simulink model "generic_20250508_0051_updated"  (R2024a)
settings: Solver=FixedStepDiscrete  StartTime=0.0  StopTime=inf  FixedStep=0.001  RelTol=1e-3  EnableMultiTasking=on
undefined symbols (not defined in the file): left_first_line_point_x, right_first_line_point_x, route1_waypoint_raw
libraries: CarMaker4SL x62, slpidlib x3, simulink x1
(part 3 of 3)

== system generic_20250508_0051_updated/CarMaker/IPG Vehicle/CarAndTrailer/Forces/Vehicle Forces ==
  Sync_In : Inport
  Bus Creator1 : BusCreator  Inputs=12
  Bus Creator8 : BusCreator  Inputs=16
  BusCreator1 : BusCreator  Inputs=4
  BusCreator2 : BusCreator  Inputs=9
  Demux : Demux  Outputs=16
      settings: DisplayOption=none
  Demux1 : Demux  Outputs=12
      settings: DisplayOption=none
  Demux2 : Demux  Outputs=13
      settings: DisplayOption=none
  Forces : S-Function  FunctionName=CM_Sfun  Parameters='Forces'  SFunctionDeploymentMode=off  EnableBusSupport=off
  Terminator : Terminator
  Sync_Out : Outport  VectorParamsAs1DForOutWhenUnconnected=off
  Car.Virtual : Outport  Port=2  VectorParamsAs1DForOutWhenUnconnected=off
  Car.Aero : Outport  Port=3  VectorParamsAs1DForOutWhenUnconnected=off
  Car.Load : Outport  Port=4  VectorParamsAs1DForOutWhenUnconnected=off
  wires:
  BusCreator1/1 -> Terminator/1  "Aero IF (in)"
  Demux2/13 -> BusCreator2/9  "car Aero Trq_1 z"
  Demux2/12 -> BusCreator2/8  "car Aero Trq_1 y"
  Demux2/11 -> BusCreator2/7  "car Aero Trq_1 x"
  Demux2/10 -> BusCreator2/6  "car Aero Frc_1 z"
  Demux2/9 -> BusCreator2/5  "car Aero Frc_1 y"
  Demux2/8 -> BusCreator2/4  "car Aero Frc_1 x"
  Demux2/7 -> BusCreator2/3  "car Aero PoA_1 z"
  Demux2/6 -> BusCreator2/2  "car Aero PoA_1 y"
  Demux2/5 -> BusCreator2/1  "car Aero PoA_1 x"
  Demux2/4 -> BusCreator1/4  "car Aero tau_1"
  Demux2/3 -> BusCreator1/3  "car Aero ApproachVel_1 z"
  Demux2/2 -> BusCreator1/2  "car Aero ApproachVel_1 y"
  Demux2/1 -> BusCreator1/1  "car Aero ApproachVel_1 x"
  Demux/16 -> Bus Creator8/16  "Car Load_3 tz"
  Demux/15 -> Bus Creator8/15  "Car Load_3 ty"
  Demux/14 -> Bus Creator8/14  "Car Load_3 tx"
  Demux/13 -> Bus Creator8/13  "Car Load_3 mass"
  Demux1/12 -> Bus Creator1/12  "Car Virtual Trq_0 z"
  Demux1/11 -> Bus Creator1/11  "Car Virtual Trq_0 y"
  Demux1/10 -> Bus Creator1/10  "Car Virtual Trq_0 x"
  Demux1/9 -> Bus Creator1/9  "Car Virtual Trq_1 z"
  Demux1/8 -> Bus Creator1/8  "Car Virtual Trq_1 y"
  Demux1/7 -> Bus Creator1/7  "Car Virtual Trq_1 x"
  Demux1/6 -> Bus Creator1/6  "Car Virtual Frc_0 z"
  Demux1/5 -> Bus Creator1/5  "Car Virtual Frc_0 y"
  Demux1/4 -> Bus Creator1/4  "Car Virtual Frc_0 x"
  Sync_In/1 -> Forces/1
  Forces/1 -> Sync_Out/1
  BusCreator2/1 -> Car.Aero/1
  Demux1/1 -> Bus Creator1/1  "Car Virtual Frc_1 x"
  Demux1/2 -> Bus Creator1/2  "Car Virtual Frc_1 y"
  Demux1/3 -> Bus Creator1/3  "Car Virtual Frc_1 z"
  Forces/3 -> Demux2/1
  Forces/2 -> Demux1/1
  Bus Creator1/1 -> Car.Virtual/1
  Bus Creator8/1 -> Car.Load/1
  Demux/1 -> Bus Creator8/1  "Car Load_0 mass"
  Demux/2 -> Bus Creator8/2  "Car Load_0 tx"
  Demux/3 -> Bus Creator8/3  "Car Load_0 ty"
  Demux/4 -> Bus Creator8/4  "Car Load_0 tz"
  Demux/5 -> Bus Creator8/5  "Car Load_1 mass"
  Demux/6 -> Bus Creator8/6  "Car Load_1 tx"
  Demux/7 -> Bus Creator8/7  "Car Load_1 ty"
  Demux/8 -> Bus Creator8/8  "Car Load_1 tz"
  Demux/9 -> Bus Creator8/9  "Car Load_2 mass"
  Demux/10 -> Bus Creator8/10  "Car Load_2 tx"
  Demux/11 -> Bus Creator8/11  "Car Load_2 ty"
  Demux/12 -> Bus Creator8/12  "Car Load_2 tz"
  Forces/4 -> Demux/1

== system generic_20250508_0051_updated/CarMaker/IPG Vehicle/CarAndTrailer/Trailer/CreateBus Car.Hitch.FrcTrq ==
  In1 : Inport
  Bus Creator7 : BusCreator  Inputs=6
  Demux7 : Demux  Outputs=6
      settings: DisplayOption=none
  Out1 : Outport  VectorParamsAs1DForOutWhenUnconnected=off
  wires:
  In1/1 -> Demux7/1
  Bus Creator7/1 -> Out1/1
  Demux7/6 -> Bus Creator7/6  "Car Hitch Trq2Car z"
  Demux7/5 -> Bus Creator7/5  "Car Hitch Trq2Car y"
  Demux7/4 -> Bus Creator7/4  "Car Hitch Trq2Car x"
  Demux7/3 -> Bus Creator7/3  "Car Hitch Frc2Car z"
  Demux7/2 -> Bus Creator7/2  "Car Hitch Frc2Car y"
  Demux7/1 -> Bus Creator7/1  "Car Hitch Frc2Car x"

== system generic_20250508_0051_updated/CarMaker/IPG Vehicle/CarAndTrailer/Trailer/CreateBus Vhcl.Motion ==
  In1 : Inport
  BusCreator : BusCreator  Inputs=15
  Demux : Demux  Outputs=15
      settings: DisplayOption=none
  Out1 : Outport  VectorParamsAs1DForOutWhenUnconnected=off
  wires:
  Demux/15 -> BusCreator/15  "Vhcl YawAcc"
  Demux/14 -> BusCreator/14  "Vhcl YawVel"
  Demux/13 -> BusCreator/13  "Vhcl Yaw"
  Demux/12 -> BusCreator/12  "Vhcl PitchAcc"
  Demux/11 -> BusCreator/11  "Vhcl PitchVel"
  Demux/10 -> BusCreator/10  "Vhcl Pitch"
  Demux/9 -> BusCreator/9  "Vhcl RollAcc"
  Demux/8 -> BusCreator/8  "Vhcl RollVel"
  Demux/7 -> BusCreator/7  "Vhcl Roll"
  Demux/6 -> BusCreator/6  "Vhcl Hitch_Pos z"
  Demux/5 -> BusCreator/5  "Vhcl Hitch_Pos y"
  Demux/4 -> BusCreator/4  "Vhcl Hitch_Pos x"
  Demux/3 -> BusCreator/3  "Vhcl sRoad"
  Demux/2 -> BusCreator/2  "Vhcl Distance"
  Demux/1 -> BusCreator/1  "Vhcl v"
  In1/1 -> Demux/1
  BusCreator/1 -> Out1/1

== system generic_20250508_0051_updated/CarMaker/IPG Vehicle/CarAndTrailer/Trailer/CreateBus Vhcl.PoI ==
  In1 : Inport
  Bus Creator3 : BusCreator  Inputs=18
  Demux3 : Demux  Outputs=18
      settings: DisplayOption=none
  Out1 : Outport  VectorParamsAs1DForOutWhenUnconnected=off
  wires:
  Demux3/18 -> Bus Creator3/18  "Vhcl PoI_GCS Elev"
  Demux3/17 -> Bus Creator3/17  "Vhcl PoI_GCS Lat"
  Demux3/16 -> Bus Creator3/16  "Vhcl PoI_GCS Long"
  Demux3/15 -> Bus Creator3/15  "Vhcl PoI_Acc_1 z"
  Demux3/14 -> Bus Creator3/14  "Vhcl PoI_Acc_1 y"
  Demux3/13 -> Bus Creator3/13  "Vhcl PoI_Acc_1 x"
  Demux3/12 -> Bus Creator3/12  "Vhcl PoI_Vel_1 z"
  Demux3/11 -> Bus Creator3/11  "Vhcl PoI_Vel_1 y"
  Demux3/10 -> Bus Creator3/10  "Vhcl PoI_Vel_1 x"
  Demux3/9 -> Bus Creator3/9  "Vhcl PoI_Acc z"
  Demux3/8 -> Bus Creator3/8  "Vhcl PoI_Acc y"
  Demux3/7 -> Bus Creator3/7  "Vhcl PoI_Acc x"
  Demux3/6 -> Bus Creator3/6  "Vhcl PoI_Vel z"
  Demux3/5 -> Bus Creator3/5  "Vhcl PoI_Vel y"
  Demux3/4 -> Bus Creator3/4  "Vhcl PoI_Vel x"
  Demux3/3 -> Bus Creator3/3  "Vhcl PoI_Pos z"
  Demux3/2 -> Bus Creator3/2  "Vhcl PoI_Pos y"
  In1/1 -> Demux3/1
  Bus Creator3/1 -> Out1/1
  Demux3/1 -> Bus Creator3/1  "Vhcl PoI_Pos x"

== system generic_20250508_0051_updated/CarMaker/IPG Vehicle/CarAndTrailer/Trailer/CreateBus Vhcl.Steering ==
  In1 : Inport
  Bus Creator3 : BusCreator  Inputs=4
  Demux : Demux
      settings: DisplayOption=none
  Out1 : Outport  VectorParamsAs1DForOutWhenUnconnected=off
  wires:
  Bus Creator3/1 -> Out1/1
  Demux/1 -> Bus Creator3/1  "Vhcl Steering Ang"
  Demux/3 -> Bus Creator3/3  "Vhcl Steering AngAcc"
  Demux/2 -> Bus Creator3/2  "Vhcl Steering AngVel"
  Demux/4 -> Bus Creator3/4  "Vhcl Steering Trq"
  In1/1 -> Demux/1

== system generic_20250508_0051_updated/CarMaker/IPG Vehicle/CarAndTrailer/Trailer/CreateBus Vhcl.Wheel.FL ==
  In1 : Inport
  Bus Creator3 : BusCreator  Inputs=14
  Demux3 : Demux  Outputs=14
      settings: DisplayOption=none
  Out1 : Outport  VectorParamsAs1DForOutWhenUnconnected=off
  wires:
  Demux3/14 -> Bus Creator3/14  "Vhcl Wheel FL Trq_WhlBearing"
  Demux3/13 -> Bus Creator3/13  "Vhcl Wheel FL Trq_T2W"
  Demux3/12 -> Bus Creator3/12  "Vhcl Wheel FL SideSlip"
  Demux3/11 -> Bus Creator3/11  "Vhcl Wheel FL LongSlip"
  Demux3/10 -> Bus Creator3/10  "Vhcl Wheel FL vBelt"
  Demux3/9 -> Bus Creator3/9  "Vhcl Wheel FL Fz"
  Demux3/8 -> Bus Creator3/8  "Vhcl Wheel FL Fy"
  Demux3/7 -> Bus Creator3/7  "Vhcl Wheel FL Fx"
  Demux3/6 -> Bus Creator3/6  "Vhcl Wheel FL r_zxy z"
  Demux3/5 -> Bus Creator3/5  "Vhcl Wheel FL r_zxy y"
  Demux3/4 -> Bus Creator3/4  "Vhcl Wheel FL r_zxy x"
  Demux3/3 -> Bus Creator3/3  "Vhcl Wheel FL t z"
  Demux3/2 -> Bus Creator3/2  "Vhcl Wheel FL t y"
  In1/1 -> Demux3/1
  Bus Creator3/1 -> Out1/1
  Demux3/1 -> Bus Creator3/1  "Vhcl Wheel FL t x"

== system generic_20250508_0051_updated/CarMaker/IPG Vehicle/CarAndTrailer/Trailer/CreateBus Vhcl.Wheel.FR ==
  In1 : Inport
  Bus Creator3 : BusCreator  Inputs=14
  Demux3 : Demux  Outputs=14
      settings: DisplayOption=none
  Out1 : Outport  VectorParamsAs1DForOutWhenUnconnected=off
  wires:
  Demux3/14 -> Bus Creator3/14  "Vhcl Wheel FR Trq_WhlBearing"
  Demux3/13 -> Bus Creator3/13  "Vhcl Wheel FR Trq_T2W"
  Demux3/12 -> Bus Creator3/12  "Vhcl Wheel FR SideSlip"
  Demux3/11 -> Bus Creator3/11  "Vhcl Wheel FR LongSlip"
  Demux3/10 -> Bus Creator3/10  "Vhcl Wheel FR vBelt"
  Demux3/9 -> Bus Creator3/9  "Vhcl Wheel FR Fz"
  Demux3/8 -> Bus Creator3/8  "Vhcl Wheel FR Fy"
  Demux3/7 -> Bus Creator3/7  "Vhcl Wheel FR Fx"
  Demux3/6 -> Bus Creator3/6  "Vhcl Wheel FR r_zxy z"
  Demux3/5 -> Bus Creator3/5  "Vhcl Wheel FR r_zxy y"
  Demux3/4 -> Bus Creator3/4  "Vhcl Wheel FR r_zxy x"
  Demux3/3 -> Bus Creator3/3  "Vhcl Wheel FR t z"
  Demux3/2 -> Bus Creator3/2  "Vhcl Wheel FR t y"
  In1/1 -> Demux3/1
  Bus Creator3/1 -> Out1/1
  Demux3/1 -> Bus Creator3/1  "Vhcl Wheel FR t x"

== system generic_20250508_0051_updated/CarMaker/IPG Vehicle/CarAndTrailer/Trailer/CreateBus Vhcl.Wheel.RL ==
  In1 : Inport
  Bus Creator3 : BusCreator  Inputs=14
  Demux3 : Demux  Outputs=14
      settings: DisplayOption=none
  Out1 : Outport  VectorParamsAs1DForOutWhenUnconnected=off
  wires:
  Demux3/14 -> Bus Creator3/14  "Vhcl Wheel RL Trq_WhlBearing"
  Demux3/13 -> Bus Creator3/13  "Vhcl Wheel RL Trq_T2W"
  Demux3/12 -> Bus Creator3/12  "Vhcl Wheel RL SideSlip"
  Demux3/11 -> Bus Creator3/11  "Vhcl Wheel RL LongSlip"
  Demux3/10 -> Bus Creator3/10  "Vhcl Wheel RL vBelt"
  Demux3/9 -> Bus Creator3/9  "Vhcl Wheel RL Fz"
  Demux3/8 -> Bus Creator3/8  "Vhcl Wheel RL Fy"
  Demux3/7 -> Bus Creator3/7  "Vhcl Wheel RL Fx"
  Demux3/6 -> Bus Creator3/6  "Vhcl Wheel RL r_zxy z"
  Demux3/5 -> Bus Creator3/5  "Vhcl Wheel RL r_zxy y"
  Demux3/4 -> Bus Creator3/4  "Vhcl Wheel RL r_zxy x"
  Demux3/3 -> Bus Creator3/3  "Vhcl Wheel RL t z"
  Demux3/2 -> Bus Creator3/2  "Vhcl Wheel RL t y"
  In1/1 -> Demux3/1
  Bus Creator3/1 -> Out1/1
  Demux3/1 -> Bus Creator3/1  "Vhcl Wheel RL t x"

== system generic_20250508_0051_updated/CarMaker/IPG Vehicle/CarAndTrailer/Trailer/CreateBus Vhcl.Wheel.RR ==
  In1 : Inport
  Bus Creator3 : BusCreator  Inputs=14
  Demux3 : Demux  Outputs=14
      settings: DisplayOption=none
  Out1 : Outport  VectorParamsAs1DForOutWhenUnconnected=off
  wires:
  Demux3/14 -> Bus Creator3/14  "Vhcl Wheel RR Trq_WhlBearing"
  Demux3/13 -> Bus Creator3/13  "Vhcl Wheel RR Trq_T2W"
  Demux3/12 -> Bus Creator3/12  "Vhcl Wheel RR SideSlip"
  Demux3/11 -> Bus Creator3/11  "Vhcl Wheel RR LongSlip"
  Demux3/10 -> Bus Creator3/10  "Vhcl Wheel RR vBelt"
  Demux3/9 -> Bus Creator3/9  "Vhcl Wheel RR Fz"
  Demux3/8 -> Bus Creator3/8  "Vhcl Wheel RR Fy"
  Demux3/7 -> Bus Creator3/7  "Vhcl Wheel RR Fx"
  Demux3/6 -> Bus Creator3/6  "Vhcl Wheel RR r_zxy z"
  Demux3/5 -> Bus Creator3/5  "Vhcl Wheel RR r_zxy y"
  Demux3/4 -> Bus Creator3/4  "Vhcl Wheel RR r_zxy x"
  Demux3/3 -> Bus Creator3/3  "Vhcl Wheel RR t z"
  Demux3/2 -> Bus Creator3/2  "Vhcl Wheel RR t y"
  In1/1 -> Demux3/1
  Bus Creator3/1 -> Out1/1
  Demux3/1 -> Bus Creator3/1  "Vhcl Wheel RR t x"

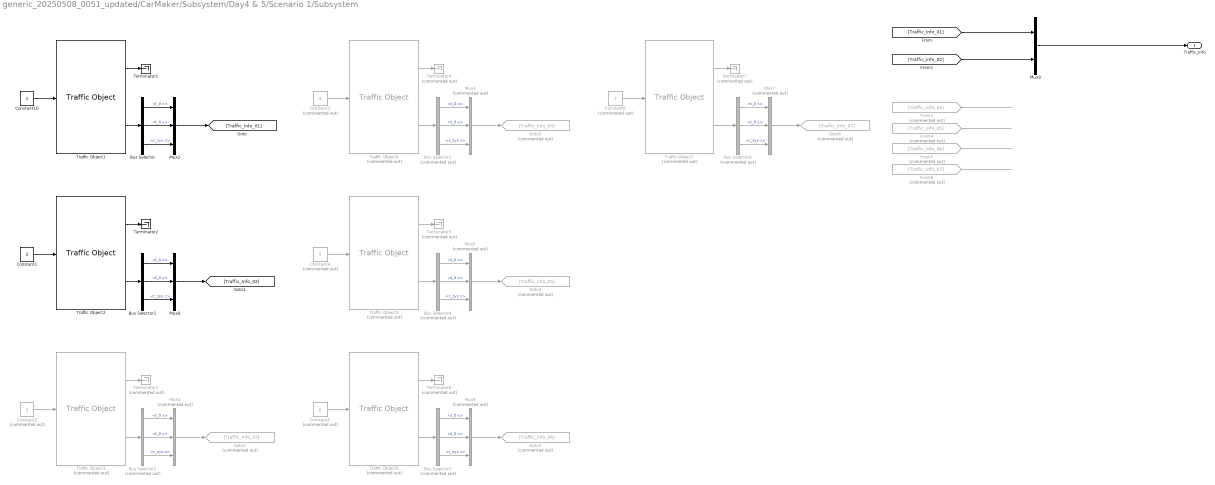
== system generic_20250508_0051_updated/CarMaker/Subsystem/Day4 & 5/Scenario 1/Subsystem ==
  Bus Selector : BusSelector  OutputSignals=t_0 x,t_0 y,r_zyx z
  Bus Selector1 : BusSelector  OutputSignals=t_0 x,t_0 y,r_zyx z
  Bus Selector{2..6} (5 alike) : BusSelector  Commented=on  OutputSignals=t_0 x,t_0 y,r_zyx z
  Constant1 : Constant  Value=2
  Constant10 : Constant
  Constant2 : Constant  Commented=on  Value=3
  Constant3 : Constant  Commented=on  Value=4
  Constant4 : Constant  Commented=on  Value=5
  Constant5 : Constant  Commented=on  Value=6
  Constant6 : Constant  Commented=on  Value=7
  From3 : From  Commented=on  GotoTag=Traffic_Info_04
  From4 : From  Commented=on  GotoTag=Traffic_Info_05
  From5 : From  Commented=on  GotoTag=Traffic_Info_06
  From6 : From  Commented=on  GotoTag=Traffic_Info_07
  Goto2 : Goto  Commented=on  GotoTag=Traffic_Info_03
  Goto3 : Goto  Commented=on  GotoTag=Traffic_Info_04
  Goto4 : Goto  Commented=on  GotoTag=Traffic_Info_05
  Goto5 : Goto  Commented=on  GotoTag=Traffic_Info_06
  Goto6 : Goto  Commented=on  GotoTag=Traffic_Info_07
  Mux2 : Mux  Inputs=3
  Mux{3..7} (5 alike) : Mux  Commented=on  Inputs=3
  Mux8 : Mux  Inputs=3
  Mux9 : Mux  Inputs=2
  Terminator1 : Terminator
  Terminator2 : Terminator
  Terminator{3..7} (5 alike) : Terminator  Commented=on
  Traffic Object1 : CarMaker4SL/Traffic Object  xname=T01  ximode=Traffic Id  xstime=Inherited
      settings: SourceProductName=CarMaker4SL
  Traffic Object2 : CarMaker4SL/Traffic Object  xname=T02  ximode=Traffic Id  xstime=Inherited
      settings: SourceProductName=CarMaker4SL
  Traffic Object3 : CarMaker4SL/Traffic Object  Commented=on  xname=T03  ximode=Traffic Id  xstime=Inherited
      settings: SourceProductName=CarMaker4SL
  Traffic Object4 : CarMaker4SL/Traffic Object  Commented=on  xname=T04  ximode=Traffic Id  xstime=Inherited
      settings: SourceProductName=CarMaker4SL
  Traffic Object5 : CarMaker4SL/Traffic Object  Commented=on  xname=T05  ximode=Traffic Id  xstime=Inherited
      settings: SourceProductName=CarMaker4SL
  Traffic Object6 : CarMaker4SL/Traffic Object  Commented=on  xname=T06  ximode=Traffic Id  xstime=Inherited
      settings: SourceProductName=CarMaker4SL
  Traffic Object7 : CarMaker4SL/Traffic Object  Commented=on  xname=T07  ximode=Traffic Id  xstime=Inherited
      settings: SourceProductName=CarMaker4SL
  Traffic_Info : Outport
  wires:
  Constant10/1 -> Traffic Object1/1
  Traffic Object1/1 -> Terminator1/1
  Traffic Object2/1 -> Terminator2/1
  Constant1/1 -> Traffic Object2/1
  Constant2/1 -> Traffic Object3/1
  Traffic Object3/1 -> Terminator3/1
  Traffic Object4/1 -> Terminator4/1
  Constant3/1 -> Traffic Object4/1
  Constant4/1 -> Traffic Object5/1
  Traffic Object5/1 -> Terminator5/1
  Traffic Object6/1 -> Terminator6/1
  Constant5/1 -> Traffic Object6/1
  Constant6/1 -> Traffic Object7/1
  Traffic Object7/1 -> Terminator7/1
  From3/1 -> ?
  From4/1 -> ?
  From5/1 -> ?
  From6/1 -> ?
  Traffic Object1/2 -> Bus Selector/1
  Bus Selector/1 -> Mux2/1  "<t_0 x>"
  Bus Selector/2 -> Mux2/2  "<t_0 y>"
  Bus Selector/3 -> Mux2/3  "<r_zyx z>"
  Bus Selector1/2 -> Mux8/2  "<t_0 y>"
  Mux8/1 -> [Traffic_Info_02]
  Bus Selector1/1 -> Mux8/1  "<t_0 x>"
  Bus Selector1/3 -> Mux8/3  "<r_zyx z>"
  Traffic Object2/2 -> Bus Selector1/1
  Bus Selector2/2 -> Mux3/2  "<t_0 y>"
  Mux3/1 -> Goto2/1
  Bus Selector2/1 -> Mux3/1  "<t_0 x>"
  Bus Selector2/3 -> Mux3/3  "<r_zyx z>"
  Traffic Object3/2 -> Bus Selector2/1
  Bus Selector3/2 -> Mux4/2  "<t_0 y>"
  Mux4/1 -> Goto3/1
  Bus Selector3/1 -> Mux4/1  "<t_0 x>"
  Bus Selector3/3 -> Mux4/3  "<r_zyx z>"
  Traffic Object4/2 -> Bus Selector3/1
  Bus Selector4/2 -> Mux5/2  "<t_0 y>"
  Mux5/1 -> Goto4/1
  Bus Selector4/1 -> Mux5/1  "<t_0 x>"
  Bus Selector4/3 -> Mux5/3  "<r_zyx z>"
  Traffic Object5/2 -> Bus Selector4/1
  Bus Selector5/2 -> Mux6/2  "<t_0 y>"
  Mux6/1 -> Goto5/1
  Bus Selector5/1 -> Mux6/1  "<t_0 x>"
  Bus Selector5/3 -> Mux6/3  "<r_zyx z>"
  Traffic Object6/2 -> Bus Selector5/1
  Bus Selector6/2 -> Mux7/2  "<t_0 y>"
  Mux7/1 -> Goto6/1
  Bus Selector6/1 -> Mux7/1  "<t_0 x>"
  Bus Selector6/3 -> Mux7/3  "<r_zyx z>"
  Traffic Object7/2 -> Bus Selector6/1
  Mux2/1 -> [Traffic_Info_01]
  [Traffic_Info_01] -> Mux9/1
  [Traffic_Info_02] -> Mux9/2
  Mux9/1 -> Traffic_Info/1

== system generic_20250508_0051_updated/CarMaker/IPG Vehicle/CarAndTrailer/Forces/Suspension Forces/Suspension External Forces Update ==
  Bus Creator21 : BusCreator  Inputs=6
  Bus Creator22 : BusCreator  Inputs=4
  Bus Creator23 : BusCreator  Inputs=4
  From : From  TagVisibility=global
  Ground{32..39} (8 alike) : Ground
  Out1 : Outport
  wires:
  [D] -> Bus Creator21/4
  Ground36/1 -> Bus Creator22/1
  From/1 -> Bus Creator21/1
  [B] -> Bus Creator21/2
  Ground34/1 -> Bus Creator23/3
  Ground32/1 -> Bus Creator23/1
  [C] -> Bus Creator21/3
  Bus Creator23/1 -> Bus Creator21/5
  Ground33/1 -> Bus Creator23/2
  Bus Creator22/1 -> Bus Creator21/6
  Bus Creator21/1 -> Out1/1
  Ground35/1 -> Bus Creator23/4
  Ground39/1 -> Bus Creator22/4
  Ground38/1 -> Bus Creator22/3
  Ground37/1 -> Bus Creator22/2

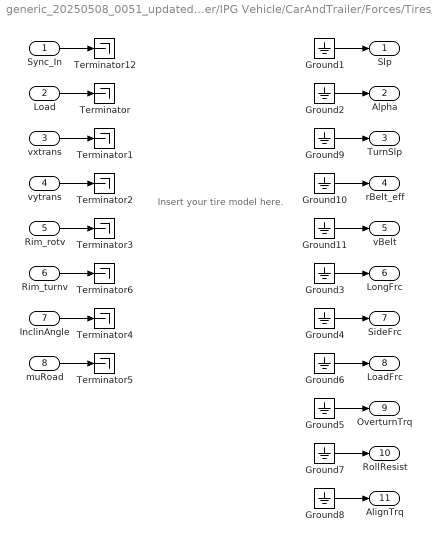
== system generic_20250508_0051_updated/CarMaker/IPG Vehicle/CarAndTrailer/Forces/Tires/TireFL ==
  note: Insert your tire model here.
  Sync_In : Inport
  Load : Inport  Port=2
  vxtrans : Inport  Port=3
  vytrans : Inport  Port=4
  Rim_rotv : Inport  Port=5
  Rim_turnv : Inport  Port=6
  InclinAngle : Inport  Port=7
  muRoad : Inport  Port=8
  Ground{1..11} (11 alike) : Ground
  Terminator{,1..6,12} (8 alike) : Terminator
  Slp : Outport  VectorParamsAs1DForOutWhenUnconnected=off
  Alpha : Outport  Port=2  VectorParamsAs1DForOutWhenUnconnected=off
  TurnSlp : Outport  Port=3  VectorParamsAs1DForOutWhenUnconnected=off
  rBelt_eff : Outport  Port=4  VectorParamsAs1DForOutWhenUnconnected=off
  vBelt : Outport  Port=5  VectorParamsAs1DForOutWhenUnconnected=off
  LongFrc : Outport  Port=6  VectorParamsAs1DForOutWhenUnconnected=off
  SideFrc : Outport  Port=7  VectorParamsAs1DForOutWhenUnconnected=off
  LoadFrc : Outport  Port=8  VectorParamsAs1DForOutWhenUnconnected=off
  OverturnTrq : Outport  Port=9  VectorParamsAs1DForOutWhenUnconnected=off
  RollResist : Outport  Port=10  VectorParamsAs1DForOutWhenUnconnected=off
  AlignTrq : Outport  Port=11  VectorParamsAs1DForOutWhenUnconnected=off
  wires:
  Ground11/1 -> vBelt/1
  Ground10/1 -> rBelt_eff/1
  Ground9/1 -> TurnSlp/1
  Rim_turnv/1 -> Terminator6/1
  Sync_In/1 -> Terminator12/1
  Ground2/1 -> Alpha/1
  Ground3/1 -> LongFrc/1
  Ground4/1 -> SideFrc/1
  Ground5/1 -> OverturnTrq/1
  vxtrans/1 -> Terminator1/1
  vytrans/1 -> Terminator2/1
  Rim_rotv/1 -> Terminator3/1
  InclinAngle/1 -> Terminator4/1
  muRoad/1 -> Terminator5/1
  Load/1 -> Terminator/1
  Ground1/1 -> Slp/1
  Ground6/1 -> LoadFrc/1
  Ground7/1 -> RollResist/1
  Ground8/1 -> AlignTrq/1

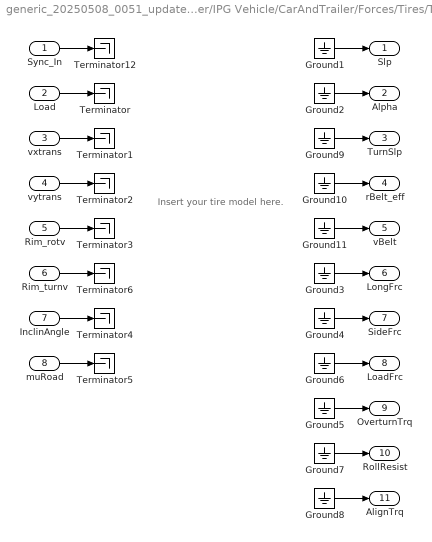
== system generic_20250508_0051_updated/CarMaker/IPG Vehicle/CarAndTrailer/Forces/Tires/TireFR ==
  note: Insert your tire model here.
  Sync_In : Inport
  Load : Inport  Port=2
  vxtrans : Inport  Port=3
  vytrans : Inport  Port=4
  Rim_rotv : Inport  Port=5
  Rim_turnv : Inport  Port=6
  InclinAngle : Inport  Port=7
  muRoad : Inport  Port=8
  Ground{1..11} (11 alike) : Ground
  Terminator{,1..6,12} (8 alike) : Terminator
  Slp : Outport  VectorParamsAs1DForOutWhenUnconnected=off
  Alpha : Outport  Port=2  VectorParamsAs1DForOutWhenUnconnected=off
  TurnSlp : Outport  Port=3  VectorParamsAs1DForOutWhenUnconnected=off
  rBelt_eff : Outport  Port=4  VectorParamsAs1DForOutWhenUnconnected=off
  vBelt : Outport  Port=5  VectorParamsAs1DForOutWhenUnconnected=off
  LongFrc : Outport  Port=6  VectorParamsAs1DForOutWhenUnconnected=off
  SideFrc : Outport  Port=7  VectorParamsAs1DForOutWhenUnconnected=off
  LoadFrc : Outport  Port=8  VectorParamsAs1DForOutWhenUnconnected=off
  OverturnTrq : Outport  Port=9  VectorParamsAs1DForOutWhenUnconnected=off
  RollResist : Outport  Port=10  VectorParamsAs1DForOutWhenUnconnected=off
  AlignTrq : Outport  Port=11  VectorParamsAs1DForOutWhenUnconnected=off
  wires:
  Ground11/1 -> vBelt/1
  Ground10/1 -> rBelt_eff/1
  Ground9/1 -> TurnSlp/1
  Rim_turnv/1 -> Terminator6/1
  Sync_In/1 -> Terminator12/1
  Ground2/1 -> Alpha/1
  Ground3/1 -> LongFrc/1
  Ground4/1 -> SideFrc/1
  Ground5/1 -> OverturnTrq/1
  vxtrans/1 -> Terminator1/1
  vytrans/1 -> Terminator2/1
  Rim_rotv/1 -> Terminator3/1
  InclinAngle/1 -> Terminator4/1
  muRoad/1 -> Terminator5/1
  Load/1 -> Terminator/1
  Ground1/1 -> Slp/1
  Ground6/1 -> LoadFrc/1
  Ground7/1 -> RollResist/1
  Ground8/1 -> AlignTrq/1

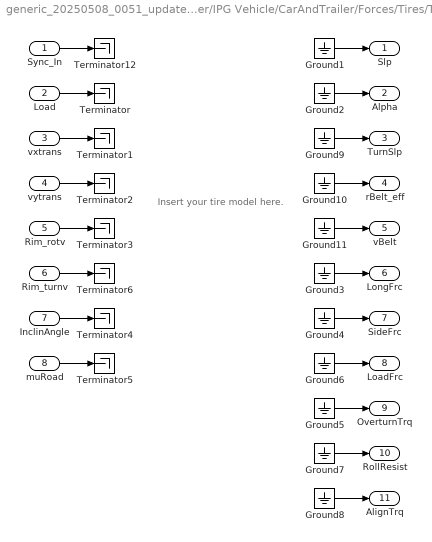
== system generic_20250508_0051_updated/CarMaker/IPG Vehicle/CarAndTrailer/Forces/Tires/TireRL ==
  note: Insert your tire model here.
  Sync_In : Inport
  Load : Inport  Port=2
  vxtrans : Inport  Port=3
  vytrans : Inport  Port=4
  Rim_rotv : Inport  Port=5
  Rim_turnv : Inport  Port=6
  InclinAngle : Inport  Port=7
  muRoad : Inport  Port=8
  Ground{1..11} (11 alike) : Ground
  Terminator{,1..6,12} (8 alike) : Terminator
  Slp : Outport  VectorParamsAs1DForOutWhenUnconnected=off
  Alpha : Outport  Port=2  VectorParamsAs1DForOutWhenUnconnected=off
  TurnSlp : Outport  Port=3  VectorParamsAs1DForOutWhenUnconnected=off
  rBelt_eff : Outport  Port=4  VectorParamsAs1DForOutWhenUnconnected=off
  vBelt : Outport  Port=5  VectorParamsAs1DForOutWhenUnconnected=off
  LongFrc : Outport  Port=6  VectorParamsAs1DForOutWhenUnconnected=off
  SideFrc : Outport  Port=7  VectorParamsAs1DForOutWhenUnconnected=off
  LoadFrc : Outport  Port=8  VectorParamsAs1DForOutWhenUnconnected=off
  OverturnTrq : Outport  Port=9  VectorParamsAs1DForOutWhenUnconnected=off
  RollResist : Outport  Port=10  VectorParamsAs1DForOutWhenUnconnected=off
  AlignTrq : Outport  Port=11  VectorParamsAs1DForOutWhenUnconnected=off
  wires:
  Ground11/1 -> vBelt/1
  Ground10/1 -> rBelt_eff/1
  Ground9/1 -> TurnSlp/1
  Rim_turnv/1 -> Terminator6/1
  Sync_In/1 -> Terminator12/1
  Ground2/1 -> Alpha/1
  Ground3/1 -> LongFrc/1
  Ground4/1 -> SideFrc/1
  Ground5/1 -> OverturnTrq/1
  vxtrans/1 -> Terminator1/1
  vytrans/1 -> Terminator2/1
  Rim_rotv/1 -> Terminator3/1
  InclinAngle/1 -> Terminator4/1
  muRoad/1 -> Terminator5/1
  Load/1 -> Terminator/1
  Ground1/1 -> Slp/1
  Ground6/1 -> LoadFrc/1
  Ground7/1 -> RollResist/1
  Ground8/1 -> AlignTrq/1

== system generic_20250508_0051_updated/CarMaker/IPG Vehicle/CarAndTrailer/Forces/Tires/TireRR ==
  note: Insert your tire model here.
  Sync_In : Inport
  Load : Inport  Port=2
  vxtrans : Inport  Port=3
  vytrans : Inport  Port=4
  Rim_rotv : Inport  Port=5
  Rim_turnv : Inport  Port=6
  InclinAngle : Inport  Port=7
  muRoad : Inport  Port=8
  Ground{1..11} (11 alike) : Ground
  Terminator{,1..6,12} (8 alike) : Terminator
  Slp : Outport  VectorParamsAs1DForOutWhenUnconnected=off
  Alpha : Outport  Port=2  VectorParamsAs1DForOutWhenUnconnected=off
  TurnSlp : Outport  Port=3  VectorParamsAs1DForOutWhenUnconnected=off
  rBelt_eff : Outport  Port=4  VectorParamsAs1DForOutWhenUnconnected=off
  vBelt : Outport  Port=5  VectorParamsAs1DForOutWhenUnconnected=off
  LongFrc : Outport  Port=6  VectorParamsAs1DForOutWhenUnconnected=off
  SideFrc : Outport  Port=7  VectorParamsAs1DForOutWhenUnconnected=off
  LoadFrc : Outport  Port=8  VectorParamsAs1DForOutWhenUnconnected=off
  OverturnTrq : Outport  Port=9  VectorParamsAs1DForOutWhenUnconnected=off
  RollResist : Outport  Port=10  VectorParamsAs1DForOutWhenUnconnected=off
  AlignTrq : Outport  Port=11  VectorParamsAs1DForOutWhenUnconnected=off
  wires:
  Ground11/1 -> vBelt/1
  Ground10/1 -> rBelt_eff/1
  Ground9/1 -> TurnSlp/1
  Rim_turnv/1 -> Terminator6/1
  Sync_In/1 -> Terminator12/1
  Ground2/1 -> Alpha/1
  Ground3/1 -> LongFrc/1
  Ground4/1 -> SideFrc/1
  Ground5/1 -> OverturnTrq/1
  vxtrans/1 -> Terminator1/1
  vytrans/1 -> Terminator2/1
  Rim_rotv/1 -> Terminator3/1
  InclinAngle/1 -> Terminator4/1
  muRoad/1 -> Terminator5/1
  Load/1 -> Terminator/1
  Ground1/1 -> Slp/1
  Ground6/1 -> LoadFrc/1
  Ground7/1 -> RollResist/1
  Ground8/1 -> AlignTrq/1

== matlab function generic_20250508_0051_updated/CarMaker/Subsystem/Final Project/Scenario 1/MATLAB Function1 ==
  settings: sampleTime=0.1
  data: u1 input; y output; u2 input
function y = longitudinal_speed_pd_controller_(u1, u2)
    y = 0;
end

== matlab function generic_20250508_0051_updated/CarMaker/Subsystem/Day3/Scenario 1/MATLAB Function4  ==
  settings: sampleTime=0.1
  data: waypoints_x input; waypoints_y input; local_waypoints_ output; vehicle_position input; head input; qual input; ego_idx_out output; ego_valid output
function [local_waypoints_,ego_idx_out,ego_valid]  = global_to_local_waypoints(waypoints_x,waypoints_y, vehicle_position, head, qual)
    [local_waypoints_,ego_idx_out,ego_valid] = deal(0);
end

== matlab function generic_20250508_0051_updated/CarMaker/Subsystem/Day3/Scenario 1/MATLAB Function4 1 ==
  settings: sampleTime=0.1
  data: waypoints_x input; waypoints_y input; local_waypoints_ output; vehicle_position input; head input; qual input; ego_idx_out output; ego_valid output
function [local_waypoints_,ego_idx_out,ego_valid]  = global_to_local_waypoints(waypoints_x,waypoints_y, vehicle_position, head, qual)
    [local_waypoints_,ego_idx_out,ego_valid] = deal(0);
end

== matlab function generic_20250508_0051_updated/CarMaker/Subsystem/Day2/Scenario 2 & 3/MATLAB Function1 ==
  settings: sampleTime=0.05
  data: ego_velocity input; desired_ax output; clearance input
function desired_ax = longitudinal_variant_space_pd_controller_(ego_velocity, clearance)
    desired_ax = 0;
end

== matlab function generic_20250508_0051_updated/CarMaker/Subsystem/Final Project/Scenario 1/MATLAB Function2 ==
  settings: sampleTime=0.1
  data: u input; y output
function y = lateral_pid_controller_(u)
    y = 0;
end

== matlab function generic_20250508_0051_updated/CarMaker/Subsystem/Day4 & 5/Scenario 1/MATLAB Function1 ==
  settings: sampleTime=0.05
  data: map_boundary input; mapMatrix output size=[1000, 1000]; traffic_info input; traffic_size input
function mapMatrix = generate_map_(map_boundary, traffic_info, traffic_size)
    mapMatrix = 0;
end

== matlab function generic_20250508_0051_updated/CarMaker/Subsystem/Day4 & 5/Scenario 1/MATLAB Function2 ==
  settings: sampleTime=0.1
  data: map input; y output; traffic_info input; traffic_size input
function y = add_obstacle_(map, traffic_info, traffic_size)
    y = 0;
end

== matlab function generic_20250508_0051_updated/CarMaker/Subsystem/Day6/Scenario 1/MATLAB Function1 ==
  settings: sampleTime=0.1
  data: u1 input; y output; u2 input
function y = longitudinal_speed_pd_controller_(u1, u2)
    y = 0;
end

== matlab function generic_20250508_0051_updated/CarMaker/Subsystem/Day6/Scenario 1/MATLAB Function2 ==
  settings: sampleTime=0.1
  data: u input; y output
function y = lateral_pid_controller_(u)
    y = 0;
end

== matlab function generic_20250508_0051_updated/CarMaker/Subsystem/Day1/Scenario 2/MATLAB Function4 ==
  settings: sampleTime=0.05
  data: u input; y output
function y = kalman_filter_(u)
    y = 0;
end

== matlab function generic_20250508_0051_updated/CarMaker/Subsystem/Day1/Scenario 2/MATLAB Function5 ==
  settings: sampleTime=0.05
  data: u input; y output
function y = average_filter_(u)
    y = 0;
end

== matlab function generic_20250508_0051_updated/CarMaker/Subsystem/Day1/Scenario 2/MATLAB Function6 ==
  settings: sampleTime=0.05
  data: u input; y output
function y = lowpass_filter_(u)
    y = 0;
end

== matlab function generic_20250508_0051_updated/CarMaker/Subsystem/Day3/Scenario 1/MATLAB Function4 2 ==
  settings: sampleTime=0.1
  data: local_waypoints input; poly_coeff output; x_local output; y_local output
function [poly_coeff,x_local,y_local] = fit_polynomial_to_waypoints(local_waypoints)
    [poly_coeff,x_local,y_local] = deal(0);
end

== matlab function generic_20250508_0051_updated/CarMaker/Subsystem/Day3/Scenario 1/MATLAB Function4 3 ==
  settings: sampleTime=0.1
  data: local_waypoints input; poly_coeff output; x_local output; y_local output
function [poly_coeff,x_local,y_local] = fit_polynomial_to_waypoints(local_waypoints)
    [poly_coeff,x_local,y_local] = deal(0);
end

== matlab function generic_20250508_0051_updated/CarMaker/Subsystem/Day3/Scenario 1/MATLAB Function4 4 ==
  settings: sampleTime=0.1
  data: coeff_L input; poly_coeff output; is_L output; is_R output; coeff_R input; qual_L input; qual_R input; ego_idx_L input; ego_idx_R input; ego_valid_L input; ego_valid_R input; state output; laneWidth output; coeff_L_out output; coeff_R_out output
function [poly_coeff,is_L,is_R,state,laneWidth,coeff_L_out,coeff_R_out] = make_line_to_path(coeff_L,coeff_R,qual_L,qual_R,ego_idx_L, ego_idx_R,ego_valid_L,ego_valid_R)
    [poly_coeff,is_L,is_R,state,laneWidth,coeff_L_out,coeff_R_out] = deal(0);
end

== matlab function generic_20250508_0051_updated/CarMaker/Subsystem/Day3/Scenario 1/MATLAB Function4 5 ==
  settings: sampleTime=0.1
  data: poly_coeff input; lateral_error output; x_lookahead output; velocity input; lookahead_time input
function [lateral_error,x_lookahead] = compute_lateral_error(poly_coeff, velocity, lookahead_time)
    [lateral_error,x_lookahead] = deal(0);
end

== matlab function generic_20250508_0051_updated/CarMaker/Subsystem/Day1/Scenario 1/MATLAB Function1 ==
  settings: sampleTime=0.05
  data: u input; y output
function y = kalman_filter_(u)
    y = 0;
end

== matlab function generic_20250508_0051_updated/CarMaker/Subsystem/Day3/Scenario 2/MATLAB Function4  ==
  settings: sampleTime=0.1
  data: waypoints_x input; waypoints_y input; local_point output; vehicle_position input; head input; dist output
function [local_point,dist]  = global_to_local_waypoints(waypoints_x,waypoints_y, vehicle_position, head)
    [local_point,dist] = deal(0);
end

== matlab function generic_20250508_0051_updated/CarMaker/Subsystem/Day3/Scenario 2/MATLAB Function4 1 ==
  settings: sampleTime=0.1
  data: ego_pos input; ego_heading input; steering_angle output; target_pos input; target_yaw input; Vx_target input; dt input
function steering_angle = follow_target(ego_pos, ego_heading, target_pos, target_yaw, Vx_target, dt)
    steering_angle = 0;
end

== matlab function generic_20250508_0051_updated/CarMaker/Subsystem/Day1/Scenario 1/MATLAB Function2 ==
  settings: sampleTime=0.05
  data: u input; y output
function y = average_filter_(u)
    y = 0;
end

== matlab function generic_20250508_0051_updated/CarMaker/Subsystem/Day2/Scenario 4 & 5/MATLAB Function1 ==
  settings: sampleTime=0.05
  data: poly_coeff input; lateral_error output; velocity input; lookahead_time input; x_lookahead output
function [lateral_error,x_lookahead] = compute_lateral_error(poly_coeff, velocity, lookahead_time)
    lateral_error = 0;
    x_lookahead = 0;
end

== matlab function generic_20250508_0051_updated/CarMaker/Subsystem/Day1/Scenario 1/MATLAB Function3 ==
  settings: sampleTime=0.05
  data: u input; y output
function y = lowpass_filter_(u)
    y = 0;
end

== matlab function generic_20250508_0051_updated/CarMaker/Subsystem/Day2/Scenario 4 & 5/MATLAB Function3 ==
  settings: sampleTime=0.05
  data: local_waypoints input; poly_coeff output
function poly_coeff = fit_polynomial_to_waypoints(local_waypoints)
    poly_coeff = 0;
end

== matlab function generic_20250508_0051_updated/CarMaker/Subsystem/Day2/Scenario 4 & 5/MATLAB Function4  ==
  settings: sampleTime=0.05
  data: waypoints input; local_waypoints_ output; vehicle_position input; head input
function local_waypoints_ = global_to_local_waypoints(waypoints, vehicle_position, head)
    local_waypoints_ = 0;
end

== matlab function generic_20250508_0051_updated/CarMaker/Subsystem/Day1/Scenario 3 & 4/MATLAB Function2 ==
  settings: sampleTime=0.05
  data: cross_track_error input; tire_angle output
function tire_angle = lateral_pd_controller_(cross_track_error)
    tire_angle = 0;
end

== matlab function generic_20250508_0051_updated/CarMaker/Subsystem/Day2/Scenario 1/MATLAB Function2 ==
  settings: sampleTime=0.05
  data: target_velocity input; desired_ax output; ego_velocity input
function desired_ax = longitudinal_speed_pd_controller_(target_velocity, ego_velocity)
    desired_ax = 0;
end

== matlab function generic_20250508_0051_updated/CarMaker/Subsystem/Day2/Scenario 2 & 3/MATLAB Function2 ==
  settings: sampleTime=0.05
  data: target_distance input; desired_ax output; clearance input
function desired_ax = longitudinal_space_pid_controller_(target_distance, clearance)
    desired_ax = 0;
end

== stateflow chart generic_20250508_0051_updated/CarMaker/Subsystem/Day3/Chart ==
  (default) -> (junction 1)
  (junction 1) -> (junction 3) [order 1] : [i<99]
      | {i = i + 1;}
  (junction 1) -> (junction 7) [order 2] : {i=0;}
  (junction 3) -> (junction 5)
  (junction 5) -> (junction 7)
  (junction 7) -> (junction 10)
  (junction 10) -> (junction 12) [order 1] : [i > 50]
      | {do_Logic;}
  (junction 10) -> (junction 18) [order 2]
  (junction 12) -> (junction 16)
  (junction 16) -> (junction 18)
  (junction 18) -> (junction 21)
  data: i local =0
  events: do_Logic output FUNCTION_CALL_EVENT
